simulink model "s_torsion"  (R2024a)
settings: Solver=ode1  StartTime=0.0  StopTime=5  FixedStep=0.002  RelTol=1e-3  EnableMultiTasking=on
values from neighbouring files (symbols this model uses):
  A = [0, 0, 1, 0 ... (first row only)    [Torsion_1D_ABCD_eqns_student.m]
  B = Kg * eta_g * kt * eta_m * B / Rm    [Torsion_1D_ABCD_eqns_student.m]
  C = [1, 0, 0, 0 ... (first row only)    [Torsion_1D_ABCD_eqns_student.m]    (also in pid_design.m = pid(Kp, Ki, Kd))
  D = [0; 0]    [Torsion_1D_ABCD_eqns_student.m]    (also in pid_design.m = [0])
  K = db2mag(12.15)    [pid_design.m]    (also in setup_torsion.m = d_torsion_1d_lqr(A,B))
  wcf = 2 * pi * 50.0    (= 314.159265359)    [setup_torsion.m]
  zetaf = 0.9    [setup_torsion.m]
undefined symbols (not defined in the file or in its folder): qc_get_step_size
libraries: simulink_extras x3, quarc_library x2
settings Model: ExtModeTrigDuration=5000  Creator=MLevis  LastModifiedBy=quarc_user
settings SolverCC: AlgebraicLoopSolver=TrustRegion  PositivePriorityOrder=on
settings DataIOCC: LimitDataPoints=on  SaveFormat=Array  SignalLoggingSaveFormat=ModelDataLogs  ReturnWorkspaceOutputs=off
settings OptimizationCC: ExpressionDepthLimit=2147483647  InitFltsAndDblsToZero=on
settings DebuggingCC: SaveWithParameterizedLinksMsg=none  UnderspecifiedInitializationDetection=Classic  MergeDetectMultiDrivingBlocksExec=none  SolverPrmCheckMsg=warning  FcnCallInpInsideContextMsg=warning  UnconnectedInputMsg=warning  UnconnectedOutputMsg=warning  UnconnectedLineMsg=warning  StateNameClashWarn=warning  SFUnexpectedBacktrackingDiag=warning  SFNoUnconditionalDefaultTransitionDiag=warning  SFExecutionAtInitializationDiag=none  ArithmeticOperatorsInVariantConditions=warning
settings ModelReferenceCC: PropagateSignalLabelsOutOfModel=off
settings SFSimCC: SimUseLocalCustomCode=off  CustomCodeUndefinedFunction=UseInterfaceOnly
settings RTWCC: Description=QUARC Win64 Target Using Toolchain  SystemTargetFile=quarc_win64.tlc  TemplateMakefile=quarc_default_tmf  RTWUseLocalCustomCode=off  Toolchain=QUARC win64 | nmake (64-bit Windows)  BuildConfiguration=Faster Runs  GPUComputeCapability=3.5
settings CodeAppCC: StateflowObjectComments=on
settings STFCustomTargetCC: TargetLangStandard=C89/C90 (ANSI)  ConcurrentExecutionCompliant=on  SystemTargetFile=quarc_win64.tlc
settings GRTTargetCC: TargetLangStandard=C89/C90 (ANSI)  ParMdlRefBuildCompliant=off  CompOptLevelCompliant=off  CombineOutputUpdateFcns=off  MatFileLogging=off  CPPClassGenCompliant=off  GRTInterface=on  ExtMode=on  ExtModeMexFile=quarc_comm
settings ConfigComp: CovMetricSettings=dw  CovSaveCumulativeToWorkspaceVar=on  CovSaveSingleToWorkspaceVar=on  CovExternalEMLEnable=off

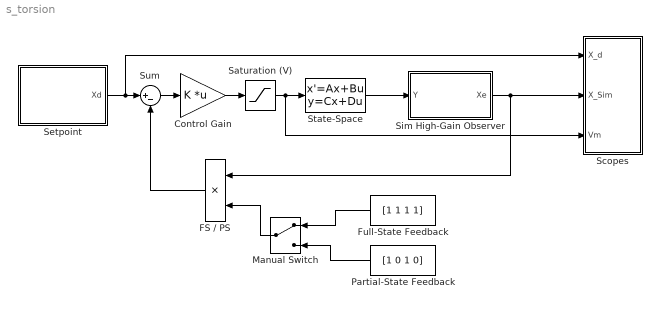
== system s_torsion ==
  Control Gain : Gain  Gain=K  Multiplication=Matrix(K*u)  SaturateOnIntegerOverflow=on  OutDataTypeStr=Inherit: Same as input  ParamDataTypeStr=Inherit: Same as input
  FS / PS : Product  RndMeth=Zero
  Full-State Feedback : Constant  Value=[1 1 1 1]
  Manual Switch : ManualSwitch
  Partial-State Feedback : Constant  Value=[1 0 1 0]
  Saturation (V) : Saturate  UpperLimit=10  LowerLimit=-10
  Scopes : Subsystem
  Setpoint : Subsystem
  Sim High-Gain Observer : Subsystem
  State-Space : StateSpace  A=A  B=B  C=C  D=D  InitialCondition=0
  Sum : Sum  Inputs=|+-
  wires:
  State-Space/1 -> Sim High-Gain Observer/1(Y)
  Full-State Feedback/1 -> Manual Switch/1
  Control Gain/1 -> Saturation (V)/1
  Partial-State Feedback/1 -> Manual Switch/2
  Manual Switch/1 -> FS / PS/2
  Sum/1 -> Control Gain/1
  FS / PS/1 -> Sum/2
  Setpoint/1(Xd) -> Sum/1, Scopes/1(X_d)
  Saturation (V)/1 -> State-Space/1, Scopes/3(Vm)
  Sim High-Gain Observer/1(Xe) -> Scopes/2(X_Sim), FS / PS/1

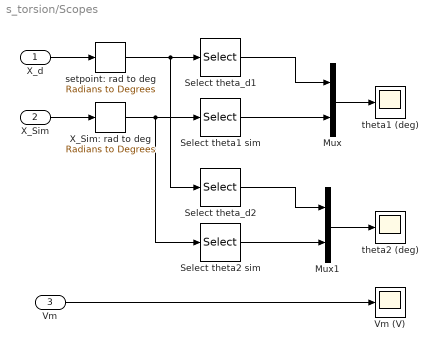
== system s_torsion/Scopes ==
  X_d : Inport
  X_Sim : Inport  Port=2
  Vm : Inport  Port=3
  Mux : Mux  Inputs=2
  Mux1 : Mux  Inputs=2
  Select theta1 sim : Selector  InputPortWidth=4  IndexOptions=Index vector (dialog)  Indices=1  OutputSizes=1
  Select theta2 sim : Selector  InputPortWidth=4  IndexOptions=Index vector (dialog)  Indices=2  OutputSizes=1
  Select theta_d1 : Selector  InputPortWidth=4  IndexOptions=Index vector (dialog)  Indices=1  OutputSizes=1
  Select theta_d2 : Selector  InputPortWidth=4  IndexOptions=Index vector (dialog)  Indices=2  OutputSizes=1
  Vm (V) : Scope
  X_Sim: rad to deg : simulink_extras/Transformations/Radians to Degrees
  setpoint: rad to deg : simulink_extras/Transformations/Radians to Degrees
  theta1 (deg) : Scope
  theta2 (deg) : Scope
  wires:
  Select theta1 sim/1 -> Mux/2
  Select theta2 sim/1 -> Mux1/2
  X_Sim: rad to deg/1 -> Select theta2 sim/1, Select theta1 sim/1
  X_Sim/1 -> X_Sim: rad to deg/1
  Select theta_d2/1 -> Mux1/1
  Select theta_d1/1 -> Mux/1
  setpoint: rad to deg/1 -> Select theta_d2/1, Select theta_d1/1
  Mux1/1 -> theta2 (deg)/1
  Vm/1 -> Vm (V)/1
  X_d/1 -> setpoint: rad to deg/1
  Mux/1 -> theta1 (deg)/1

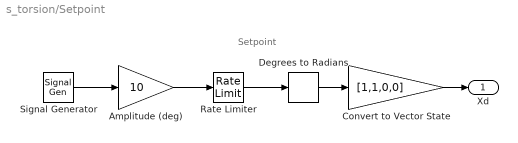
== system s_torsion/Setpoint ==
  note: Setpoint
  Amplitude (deg) : Gain  Gain=10  SaturateOnIntegerOverflow=on  OutDataTypeStr=Inherit: Same as input  ParamDataTypeStr=Inherit: Same as input
  Convert to Vector State : Gain  Gain=[1,1,0,0]
  Degrees to Radians : simulink_extras/Transformations/Degrees to Radians
  Rate Limiter : RateLimiter  RisingSlewLimit=5*180  FallingSlewLimit=-5*180  SampleTimeMode=inherited
  Signal Generator : SignalGenerator  WaveForm=square  Frequency=0.5
  Xd : Outport
  wires:
  Degrees to Radians/1 -> Convert to Vector State/1
  Rate Limiter/1 -> Degrees to Radians/1
  Amplitude (deg)/1 -> Rate Limiter/1
  Signal Generator/1 -> Amplitude (deg)/1
  Convert to Vector State/1 -> Xd/1

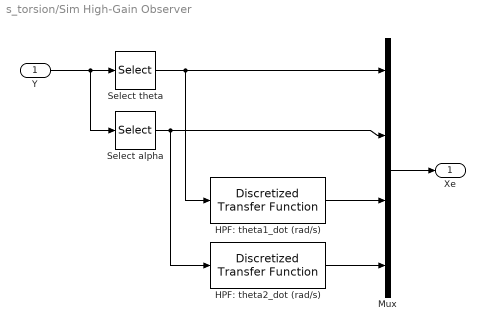
== system s_torsion/Sim High-Gain Observer ==
  Y : Inport
  HPF: theta1_dot (rad/s) : quarc_library/Discrete/Discretized Transfer Function  num=[wcf^2 0]  den=[1 2*zetaf*wcf wcf^2]  method=tustin  Ts=qc_get_step_size
      settings: SourceProductName=QUARC Targets
  HPF: theta2_dot (rad/s) : quarc_library/Discrete/Discretized Transfer Function  num=[wcf^2 0]  den=[1 2*zetaf*wcf wcf^2]  method=tustin  Ts=qc_get_step_size
      settings: SourceProductName=QUARC Targets
  Mux : Mux
  Select alpha : Selector  InputPortWidth=2  IndexOptions=Index vector (dialog)  Indices=2  OutputSizes=1
  Select theta : Selector  InputPortWidth=2  IndexOptions=Index vector (dialog)  Indices=1  OutputSizes=1
  Xe : Outport
  wires:
  Select alpha/1 -> Mux/2, HPF: theta2_dot (rad/s)/1
  Mux/1 -> Xe/1
  Y/1 -> Select alpha/1, Select theta/1
  HPF: theta1_dot (rad/s)/1 -> Mux/3
  Select theta/1 -> HPF: theta1_dot (rad/s)/1, Mux/1
  HPF: theta2_dot (rad/s)/1 -> Mux/4
